simulink library "CRYP_IM_MASTER"  (Simulink 8.6)
settings: Solver=ode45  StartTime=0.0  StopTime=10.0  RelTol=1e-3
libraries: VIS_LIB x14, cdsEpicsOut x10, cdsTP x6, cdsFiltCtrl x4, cdsMuxMatrix x4, CRYP_TM_MASTER x2, cdsFilt x2, KAGRA_UTIL x1, cdsFunctionCall x1
settings Model: Creator=controls  LastModifiedBy=controls

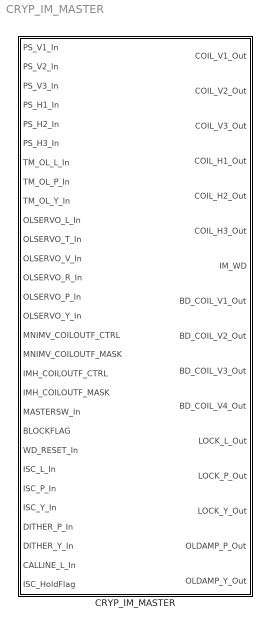
== system CRYP_IM_MASTER ==
  CRYP_IM_MASTER : Subsystem  Description=SIXOSEMSTAGE_FACE_MASTER

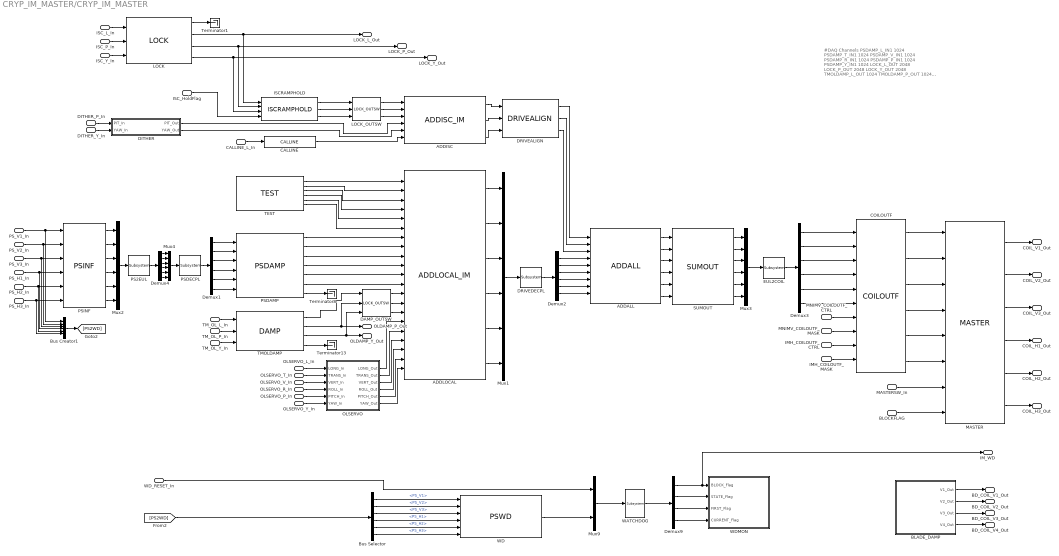
== system CRYP_IM_MASTER/CRYP_IM_MASTER ==
  note: #DAQ Channels
      | PSDAMP_L_IN1 1024
      | PSDAMP_T_IN1 1024
      | PSDAMP_V_IN1 1024
      | PSDAMP_R_IN1 1024
      | PSDAMP_P_IN1 1024
      | PSDAMP_Y_IN1 1024
      | LOCK_L_OUT 2048
      | LOCK_P_OUT 2048
      | LOCK_Y_OUT 2048
      | TMOLDAMP_L_OUT 1024
      | TMOLDAMP_P_OUT 1024
      | TMOLDAMP_Y_OUT 1024
      | PSDAMP_L_OUT 1024
      | PSDAMP_T_OUT 1024
      | PSDAMP_V_OUT 1024
      | PSDAMP_R_OUT 1024
      | PSDAMP_P_OUT 1024
      | PSDAMP_Y_OUT 1024
      | MASTER_OUT_H1 1024
      | MASTER_OUT_H2 1024
      | MASTER_OUT_H3 1024
      | MASTER_OUT_V1 1024
      | MASTER_OUT_V2 1024
      | MASTER_OUT_V3 1024
  PS_V1_In : Inport
  PS_V2_In : Inport  Port=2
  PS_V3_In : Inport  Port=3
  PS_H1_In : Inport  Port=4
  PS_H2_In : Inport  Port=5
  PS_H3_In : Inport  Port=6
  TM_OL_L_In : Inport  Port=7
  TM_OL_P_In : Inport  Port=8
  TM_OL_Y_In : Inport  Port=9
  OLSERVO_L_In : Inport  Port=10
  OLSERVO_T_In : Inport  Port=11
  OLSERVO_V_In : Inport  Port=12
  OLSERVO_R_In : Inport  Port=13
  OLSERVO_P_In : Inport  Port=14
  OLSERVO_Y_In : Inport  Port=15
  MNIMV_COILOUTF_CTRL : Inport  Port=16
  MNIMV_COILOUTF_MASK : Inport  Port=17
  IMH_COILOUTF_CTRL : Inport  Port=18
  IMH_COILOUTF_MASK : Inport  Port=19
  MASTERSW_In : Inport  Port=20
  BLOCKFLAG : Inport  Port=21
  WD_RESET_In : Inport  Port=22
  ISC_L_In : Inport  Port=23
  ISC_P_In : Inport  Port=24
  ISC_Y_In : Inport  Port=25
  DITHER_P_In : Inport  Port=26
  DITHER_Y_In : Inport  Port=27
  CALLINE_L_In : Inport  Port=28
  ISC_HoldFlag : Inport  Port=29
  ADDALL : VIS_LIB/CrypParts/ADDALL
  ADDISC : VIS_LIB/CrypParts/ADDISC_IM
  ADDLOCAL : VIS_LIB/CrypParts/ADDLOCAL_IM
  BLADE_DAMP : Subsystem
  Bus Creator1 : BusCreator  Inputs='PS_V1','PS_V2','PS_V3','PS_H1','PS_H2','PS_H3'
  Bus Selector : BusSelector  OutputSignals=PS_V1,PS_V2,PS_V3,PS_H1,PS_H2,PS_H3
  CALLINE : VIS_LIB/CALLINE
  COILOUTF : VIS_LIB/CRYp Blocks/COILOUTF
  DAMP_OUTSW : CRYP_TM_MASTER/CRYP_TM_MASTER/LOCK_OUTSW
  DITHER : Subsystem
  DRIVEALIGN : VIS_LIB/CrypParts/DRIVEALIGN
  DRIVEDECPL : cdsMuxMatrix/Subsystem  Tag=cdsMuxMatrix  Description=Any size matrix. Inputs and outputs must be connected using Mux and Demux parts.
      settings: AttributesFormatString=%<Tag>
  Demux{1..4} (4 alike) : Demux  Outputs=6
  Demux9 : Demux
  EUL2COIL : cdsMuxMatrix/Subsystem  Tag=cdsMuxMatrix  Description=Any size matrix. Inputs and outputs must be connected using Mux and Demux parts.
      settings: AttributesFormatString=%<Tag>
  ISCRAMPHOLD : KAGRA_UTIL/ISCRAMPHOLD
  LOCK : VIS_LIB/CrypParts/LOCK
  LOCK_OUTSW : CRYP_TM_MASTER/CRYP_TM_MASTER/LOCK_OUTSW
  MASTER : VIS_LIB/CRYp Blocks/MASTER
  Mux{1..4} (4 alike) : Mux  Inputs=6
  Mux9 : Mux  Inputs=2
  OLSERVO : Subsystem
  PS2EUL : cdsMuxMatrix/Subsystem  Tag=cdsMuxMatrix  Description=Any size matrix. Inputs and outputs must be connected using Mux and Demux parts.
      settings: AttributesFormatString=%<Tag>
  PSDAMP : VIS_LIB/CrypParts/PSDAMP
  PSDECPL : cdsMuxMatrix/Subsystem  Tag=cdsMuxMatrix  Description=Any size matrix. Inputs and outputs must be connected using Mux and Demux parts.
      settings: AttributesFormatString=%<Tag>
  PSINF : VIS_LIB/CrypParts/PSINF
  SUMOUT : VIS_LIB/CrypParts/SUMOUT
  TEST : VIS_LIB/CrypParts/TEST
  TMOLDAMP : VIS_LIB/CrypParts/DAMP
  Terminator1 : Terminator
  Terminator13 : Terminator
  Terminator8 : Terminator
  WATCHDOG : cdsFunctionCall/Subsystem  Tag=cdsFunctionCall  Description=inline OSEMWATCHDOG /opt/rtcds/userapps/release/vis/common/src/WATCHDOG.c
      settings: AttributesFormatString=%<Tag>\n%<Description>
  WD : VIS_LIB/CRYp Blocks/PSWD
  WDMON : Subsystem
  COIL_V1_Out : Outport
  COIL_V2_Out : Outport  Port=2
  COIL_V3_Out : Outport  Port=3
  COIL_H1_Out : Outport  Port=4
  COIL_H2_Out : Outport  Port=5
  COIL_H3_Out : Outport  Port=6
  IM_WD : Outport  Port=7
  BD_COIL_V1_Out : Outport  Port=8
  BD_COIL_V2_Out : Outport  Port=9
  BD_COIL_V3_Out : Outport  Port=10
  BD_COIL_V4_Out : Outport  Port=11
  LOCK_L_Out : Outport  Port=12
  LOCK_P_Out : Outport  Port=13
  LOCK_Y_Out : Outport  Port=14
  OLDAMP_P_Out : Outport  Port=15
  OLDAMP_Y_Out : Outport  Port=16
  wires:
  ISC_HoldFlag/1 -> ISCRAMPHOLD/4
  ISCRAMPHOLD/3 -> LOCK_OUTSW/3
  ISCRAMPHOLD/2 -> LOCK_OUTSW/2
  ISCRAMPHOLD/1 -> LOCK_OUTSW/1
  WATCHDOG/1 -> Demux9/1
  Mux9/1 -> WATCHDOG/1
  COILOUTF/3 -> MASTER/3
  COILOUTF/2 -> MASTER/2
  COILOUTF/1 -> MASTER/1
  Demux9/4 -> WDMON/4(CURRENT_Flag)
  Demux9/3 -> WDMON/3(FIRST_Flag)
  Demux9/2 -> WDMON/2(STATE_Flag)
  EUL2COIL/1 -> Demux3/1
  Mux3/1 -> EUL2COIL/1
  MASTER/6 -> COIL_H3_Out/1
  MASTER/5 -> COIL_H2_Out/1
  MASTER/4 -> COIL_H1_Out/1
  MASTER/3 -> COIL_V3_Out/1
  MASTER/2 -> COIL_V2_Out/1
  MASTER/1 -> COIL_V1_Out/1
  [PS2WD] -> Bus Selector/1
  Bus Creator1/1 -> [PS2WD]
  Mux2/1 -> PS2EUL/1
  PSINF/1 -> Mux2/1
  PSINF/2 -> Mux2/2
  PSINF/3 -> Mux2/3
  PSINF/4 -> Mux2/4
  PSINF/5 -> Mux2/5
  PSINF/6 -> Mux2/6
  Demux9/1 -> IM_WD/1, WDMON/1(BLOCK_Flag)
  MASTERSW_In/1 -> MASTER/7
  MNIMV_COILOUTF_CTRL/1 -> COILOUTF/7
  WD/1 -> Mux9/2
  WD_RESET_In/1 -> Mux9/1
  IMH_COILOUTF_CTRL/1 -> COILOUTF/9
  IMH_COILOUTF_MASK/1 -> COILOUTF/10
  PS_V3_In/1 -> Bus Creator1/3, PSINF/3
  PS_H1_In/1 -> PSINF/4, Bus Creator1/4
  PS_H2_In/1 -> Bus Creator1/5, PSINF/5
  PS_H3_In/1 -> Bus Creator1/6, PSINF/6
  PS_V1_In/1 -> Bus Creator1/1, PSINF/1
  PS_V2_In/1 -> Bus Creator1/2, PSINF/2
  MNIMV_COILOUTF_MASK/1 -> COILOUTF/8
  COILOUTF/4 -> MASTER/4
  COILOUTF/5 -> MASTER/5
  COILOUTF/6 -> MASTER/6
  ISC_L_In/1 -> LOCK/1
  ISC_P_In/1 -> LOCK/2
  ISC_Y_In/1 -> LOCK/3
  Bus Selector/6 -> WD/6  "<PS_H3>"
  Bus Selector/1 -> WD/1  "<PS_V1>"
  Bus Selector/2 -> WD/2  "<PS_V2>"
  Bus Selector/3 -> WD/3  "<PS_V3>"
  Bus Selector/4 -> WD/4  "<PS_H1>"
  Bus Selector/5 -> WD/5  "<PS_H2>"
  BLADE_DAMP/1(V1_Out) -> BD_COIL_V1_Out/1
  BLADE_DAMP/2(V2_Out) -> BD_COIL_V2_Out/1
  BLADE_DAMP/3(V3_Out) -> BD_COIL_V3_Out/1
  BLADE_DAMP/4(V4_Out) -> BD_COIL_V4_Out/1
  BLOCKFLAG/1 -> MASTER/8
  Demux3/6 -> COILOUTF/6
  Demux3/5 -> COILOUTF/5
  Demux3/4 -> COILOUTF/4
  Demux3/3 -> COILOUTF/3
  Demux3/2 -> COILOUTF/2
  Demux3/1 -> COILOUTF/1
  Demux1/1 -> PSDAMP/1
  Demux1/2 -> PSDAMP/2
  Demux1/3 -> PSDAMP/3
  Demux1/4 -> PSDAMP/4
  Demux1/5 -> PSDAMP/5
  Demux1/6 -> PSDAMP/6
  PSDAMP/7 -> Terminator8/1
  DITHER/1(PIT_Out) -> ADDISC/4
  DITHER/2(YAW_Out) -> ADDISC/5
  ADDISC/2 -> DRIVEALIGN/2
  ADDISC/1 -> DRIVEALIGN/1
  ADDISC/3 -> DRIVEALIGN/3
  TEST/6 -> ADDLOCAL/6
  TEST/5 -> ADDLOCAL/5
  TEST/4 -> ADDLOCAL/4
  TEST/3 -> ADDLOCAL/3
  TEST/2 -> ADDLOCAL/2
  TEST/1 -> ADDLOCAL/1
  PSDAMP/4 -> ADDLOCAL/10
  PSDAMP/5 -> ADDLOCAL/11
  PSDAMP/6 -> ADDLOCAL/12
  PSDAMP/1 -> ADDLOCAL/7
  PSDAMP/2 -> ADDLOCAL/8
  PSDAMP/3 -> ADDLOCAL/9
  TM_OL_L_In/1 -> TMOLDAMP/1
  TM_OL_P_In/1 -> TMOLDAMP/2
  TM_OL_Y_In/1 -> TMOLDAMP/3
  TMOLDAMP/2 -> OLDAMP_P_Out/1, DAMP_OUTSW/2
  TMOLDAMP/3 -> DAMP_OUTSW/3, OLDAMP_Y_Out/1
  TMOLDAMP/4 -> Terminator13/1
  DRIVEDECPL/1 -> Demux2/1
  Mux1/1 -> DRIVEDECPL/1
  Demux2/5 -> ADDALL/8
  Demux2/2 -> ADDALL/5
  Demux2/3 -> ADDALL/6
  Demux2/6 -> ADDALL/9
  Demux2/1 -> ADDALL/4
  Demux2/4 -> ADDALL/7
  ADDLOCAL/5 -> Mux1/5
  ADDLOCAL/4 -> Mux1/4
  ADDLOCAL/6 -> Mux1/6
  ADDLOCAL/3 -> Mux1/3
  ADDLOCAL/2 -> Mux1/2
  ADDLOCAL/1 -> Mux1/1
  DRIVEALIGN/3 -> ADDALL/3
  DRIVEALIGN/2 -> ADDALL/2
  DRIVEALIGN/1 -> ADDALL/1
  LOCK/1 -> Terminator1/1
  LOCK/4 -> LOCK_Y_Out/1, ISCRAMPHOLD/3
  LOCK/3 -> LOCK_P_Out/1, ISCRAMPHOLD/2
  LOCK/2 -> LOCK_L_Out/1, ISCRAMPHOLD/1
  DITHER_Y_In/1 -> DITHER/2(YAW_In)
  DITHER_P_In/1 -> DITHER/1(PIT_In)
  ADDALL/1 -> SUMOUT/1
  ADDALL/2 -> SUMOUT/2
  ADDALL/3 -> SUMOUT/3
  ADDALL/4 -> SUMOUT/4
  ADDALL/5 -> SUMOUT/5
  ADDALL/6 -> SUMOUT/6
  SUMOUT/1 -> Mux3/1
  SUMOUT/2 -> Mux3/2
  SUMOUT/3 -> Mux3/3
  SUMOUT/4 -> Mux3/4
  SUMOUT/5 -> Mux3/5
  SUMOUT/6 -> Mux3/6
  PSDECPL/1 -> Demux1/1
  PS2EUL/1 -> Demux4/1
  Demux4/1 -> Mux4/1
  Demux4/2 -> Mux4/2
  Demux4/3 -> Mux4/3
  Demux4/4 -> Mux4/4
  Demux4/5 -> Mux4/5
  Demux4/6 -> Mux4/6
  Mux4/1 -> PSDECPL/1
  OLSERVO_L_In/1 -> OLSERVO/1(LONG_In)
  OLSERVO_T_In/1 -> OLSERVO/2(TRANS_In)
  OLSERVO_V_In/1 -> OLSERVO/3(VERT_In)
  OLSERVO_R_In/1 -> OLSERVO/4(ROLL_In)
  OLSERVO_P_In/1 -> OLSERVO/5(PITCH_In)
  OLSERVO_Y_In/1 -> OLSERVO/6(YAW_In)
  OLSERVO/1(LONG_Out) -> ADDLOCAL/16
  OLSERVO/2(TRANS_Out) -> ADDLOCAL/17
  OLSERVO/3(VERT_Out) -> ADDLOCAL/18
  OLSERVO/4(ROLL_Out) -> ADDLOCAL/19
  OLSERVO/5(PITCH_Out) -> ADDLOCAL/20
  OLSERVO/6(YAW_Out) -> ADDLOCAL/21
  LOCK_OUTSW/1 -> ADDISC/1
  LOCK_OUTSW/2 -> ADDISC/2
  LOCK_OUTSW/3 -> ADDISC/3
  DAMP_OUTSW/1 -> ADDLOCAL/13
  DAMP_OUTSW/2 -> ADDLOCAL/14
  DAMP_OUTSW/3 -> ADDLOCAL/15
  TMOLDAMP/1 -> DAMP_OUTSW/1
  CALLINE/1 -> ADDISC/6
  CALLINE_L_In/1 -> CALLINE/1

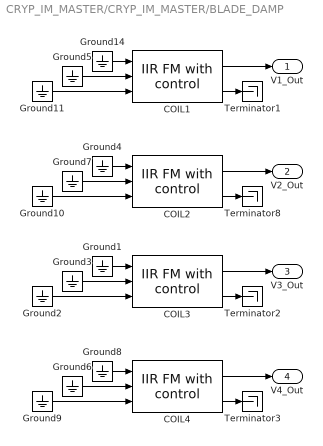
== system CRYP_IM_MASTER/CRYP_IM_MASTER/BLADE_DAMP ==
  COIL1 : cdsFiltCtrl/IIR FM with control  Tag=cdsFiltCtrl  Description=|
      | cdsFiltCntrl is the standard IIR filter module (exactly the same as cdsFilt) but with added control data output 'Ctrl'. Filter module digital signal output appears on the first output, which is called 'Val'. 'Ctrl' output has a bit pattern encoding the state of filter's on/off switches (FM1 through FM10). The bit values are:
      |                                                                                                                                                                                                                                                                                                                                       
      | module 	hex	dec                                                                                                                                                                                                                                                                                                                       
      | -----------------------                                                                                                                                                                                                                                                                                                               
      | FM1	0x20                    32                                                                                                                                                                                                                                                                                                        
      | FM2	0x80                     128                                                                                                                                                                                                                                                                                                      
      | FM3	0x200                   512                                                                                                                                                                                                                                                                                                       
      | FM4	0x800                   2048                                                                                                                                                                                                                                                                                                      
      | FM5	0x2000                 8192                                                                                                                                                                                                                                                                                                       
      | FM6	0x8000                 32768                                                                                                                                                                                                                                                                                                      
      | FM7	0x20000                131072                                                                                                                                                                                                                                                                                                     
      | FM8	0x80000                 524288                                                                                                                                                                                                                                                                                                    
      | FM9	0x200000               2097152                                                                                                                                                                                                                                                                                                    
      | FM10	0x800000               8388608                                                                                                                                                                                                                                                                                                   
      |                                                                                                                                                                                                                                                                                                                                       
      | This bit data can be used to drive some other switches or it can be output using a binary I/O module.
      settings: AttributesFormatString=%<Tag>
  COIL2 : cdsFiltCtrl/IIR FM with control  Tag=cdsFiltCtrl  Description=|
      | cdsFiltCntrl is the standard IIR filter module (exactly the same as cdsFilt) but with added control data output 'Ctrl'. Filter module digital signal output appears on the first output, which is called 'Val'. 'Ctrl' output has a bit pattern encoding the state of filter's on/off switches (FM1 through FM10). The bit values are:
      |                                                                                                                                                                                                                                                                                                                                       
      | module 	hex	dec                                                                                                                                                                                                                                                                                                                       
      | -----------------------                                                                                                                                                                                                                                                                                                               
      | FM1	0x20                    32                                                                                                                                                                                                                                                                                                        
      | FM2	0x80                     128                                                                                                                                                                                                                                                                                                      
      | FM3	0x200                   512                                                                                                                                                                                                                                                                                                       
      | FM4	0x800                   2048                                                                                                                                                                                                                                                                                                      
      | FM5	0x2000                 8192                                                                                                                                                                                                                                                                                                       
      | FM6	0x8000                 32768                                                                                                                                                                                                                                                                                                      
      | FM7	0x20000                131072                                                                                                                                                                                                                                                                                                     
      | FM8	0x80000                 524288                                                                                                                                                                                                                                                                                                    
      | FM9	0x200000               2097152                                                                                                                                                                                                                                                                                                    
      | FM10	0x800000               8388608                                                                                                                                                                                                                                                                                                   
      |                                                                                                                                                                                                                                                                                                                                       
      | This bit data can be used to drive some other switches or it can be output using a binary I/O module.
      settings: AttributesFormatString=%<Tag>
  COIL3 : cdsFiltCtrl/IIR FM with control  Tag=cdsFiltCtrl  Description=|
      | cdsFiltCntrl is the standard IIR filter module (exactly the same as cdsFilt) but with added control data output 'Ctrl'. Filter module digital signal output appears on the first output, which is called 'Val'. 'Ctrl' output has a bit pattern encoding the state of filter's on/off switches (FM1 through FM10). The bit values are:
      |                                                                                                                                                                                                                                                                                                                                       
      | module 	hex	dec                                                                                                                                                                                                                                                                                                                       
      | -----------------------                                                                                                                                                                                                                                                                                                               
      | FM1	0x20                    32                                                                                                                                                                                                                                                                                                        
      | FM2	0x80                     128                                                                                                                                                                                                                                                                                                      
      | FM3	0x200                   512                                                                                                                                                                                                                                                                                                       
      | FM4	0x800                   2048                                                                                                                                                                                                                                                                                                      
      | FM5	0x2000                 8192                                                                                                                                                                                                                                                                                                       
      | FM6	0x8000                 32768                                                                                                                                                                                                                                                                                                      
      | FM7	0x20000                131072                                                                                                                                                                                                                                                                                                     
      | FM8	0x80000                 524288                                                                                                                                                                                                                                                                                                    
      | FM9	0x200000               2097152                                                                                                                                                                                                                                                                                                    
      | FM10	0x800000               8388608                                                                                                                                                                                                                                                                                                   
      |                                                                                                                                                                                                                                                                                                                                       
      | This bit data can be used to drive some other switches or it can be output using a binary I/O module.
      settings: AttributesFormatString=%<Tag>
  COIL4 : cdsFiltCtrl/IIR FM with control  Tag=cdsFiltCtrl  Description=|
      | cdsFiltCntrl is the standard IIR filter module (exactly the same as cdsFilt) but with added control data output 'Ctrl'. Filter module digital signal output appears on the first output, which is called 'Val'. 'Ctrl' output has a bit pattern encoding the state of filter's on/off switches (FM1 through FM10). The bit values are:
      |                                                                                                                                                                                                                                                                                                                                       
      | module 	hex	dec                                                                                                                                                                                                                                                                                                                       
      | -----------------------                                                                                                                                                                                                                                                                                                               
      | FM1	0x20                    32                                                                                                                                                                                                                                                                                                        
      | FM2	0x80                     128                                                                                                                                                                                                                                                                                                      
      | FM3	0x200                   512                                                                                                                                                                                                                                                                                                       
      | FM4	0x800                   2048                                                                                                                                                                                                                                                                                                      
      | FM5	0x2000                 8192                                                                                                                                                                                                                                                                                                       
      | FM6	0x8000                 32768                                                                                                                                                                                                                                                                                                      
      | FM7	0x20000                131072                                                                                                                                                                                                                                                                                                     
      | FM8	0x80000                 524288                                                                                                                                                                                                                                                                                                    
      | FM9	0x200000               2097152                                                                                                                                                                                                                                                                                                    
      | FM10	0x800000               8388608                                                                                                                                                                                                                                                                                                   
      |                                                                                                                                                                                                                                                                                                                                       
      | This bit data can be used to drive some other switches or it can be output using a binary I/O module.
      settings: AttributesFormatString=%<Tag>
  Ground{1..11,14} (12 alike) : Ground
  Terminator{1..3,8} (4 alike) : Terminator
  V1_Out : Outport
  V2_Out : Outport  Port=2
  V3_Out : Outport  Port=3
  V4_Out : Outport  Port=4
  wires:
  COIL1/1 -> V1_Out/1
  COIL2/1 -> V2_Out/1
  COIL3/1 -> V3_Out/1
  COIL4/1 -> V4_Out/1
  Ground14/1 -> COIL1/1
  Ground5/1 -> COIL1/2
  Ground11/1 -> COIL1/3
  Ground4/1 -> COIL2/1
  Ground7/1 -> COIL2/2
  Ground10/1 -> COIL2/3
  Ground1/1 -> COIL3/1
  Ground3/1 -> COIL3/2
  Ground2/1 -> COIL3/3
  Ground8/1 -> COIL4/1
  Ground6/1 -> COIL4/2
  Ground9/1 -> COIL4/3
  COIL1/2 -> Terminator1/1
  COIL2/2 -> Terminator8/1
  COIL3/2 -> Terminator2/1
  COIL4/2 -> Terminator3/1

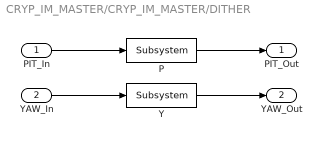
== system CRYP_IM_MASTER/CRYP_IM_MASTER/DITHER ==
  PIT_In : Inport
  YAW_In : Inport  Port=2
  P : cdsFilt/Subsystem  Tag=cdsFilt  Description=|
      | Purpose:                                                                                                                                                                                                                                  
      | Standard CDS IIR filter module.                                                                                                                                                                                                           
      |                                                                                                                                                                                                                                           
      | Operation:                                                                                                                                                                                                                                
      | Consists of 10 second order section IIR filters, plus a ramped gain stage. In FE code, also provides pre-defined test points and excitation channel inputs. The filter coefficients are defined in the LIGO system using the 'foton' tool.
      |                                                                                                                                                                                                                                           
      | Usage:                                                                                                                                                                                                                                    
      | Name the part with the desired filter module name.
      settings: AttributesFormatString=%<Tag>
  Y : cdsFilt/Subsystem  Tag=cdsFilt  Description=|
      | Purpose:                                                                                                                                                                                                                                  
      | Standard CDS IIR filter module.                                                                                                                                                                                                           
      |                                                                                                                                                                                                                                           
      | Operation:                                                                                                                                                                                                                                
      | Consists of 10 second order section IIR filters, plus a ramped gain stage. In FE code, also provides pre-defined test points and excitation channel inputs. The filter coefficients are defined in the LIGO system using the 'foton' tool.
      |                                                                                                                                                                                                                                           
      | Usage:                                                                                                                                                                                                                                    
      | Name the part with the desired filter module name.
      settings: AttributesFormatString=%<Tag>
  PIT_Out : Outport
  YAW_Out : Outport  Port=2
  wires:
  PIT_In/1 -> P/1
  Y/1 -> YAW_Out/1
  YAW_In/1 -> Y/1
  P/1 -> PIT_Out/1

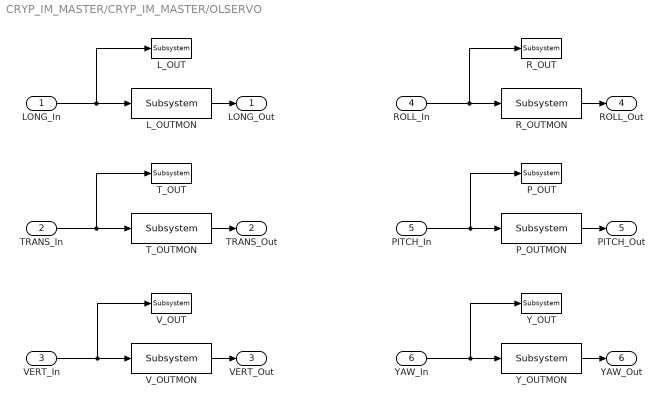
== system CRYP_IM_MASTER/CRYP_IM_MASTER/OLSERVO ==
  LONG_In : Inport
  TRANS_In : Inport  Port=2
  VERT_In : Inport  Port=3
  ROLL_In : Inport  Port=4
  PITCH_In : Inport  Port=5
  YAW_In : Inport  Port=6
  L_OUT : cdsTP/Subsystem  Tag=Test Point
      settings: AttributesFormatString=%<Tag>
  L_OUTMON : cdsEpicsOut/Subsystem  Tag=cdsEpicsOutput  Description=|
      | Purpose:                                          
      | Output a FE signal to an EPICS channel.           
      |                                                   
      | Operation:                                        
      | Takes input value and passes it to EPICS record.  
      |                                                   
      | Usage:                                            
      | Name the part with the desired EPICS rrecord name.
      settings: AttributesFormatString=%<Tag>
  P_OUT : cdsTP/Subsystem  Tag=Test Point
      settings: AttributesFormatString=%<Tag>
  P_OUTMON : cdsEpicsOut/Subsystem  Tag=cdsEpicsOutput  Description=|
      | Purpose:                                          
      | Output a FE signal to an EPICS channel.           
      |                                                   
      | Operation:                                        
      | Takes input value and passes it to EPICS record.  
      |                                                   
      | Usage:                                            
      | Name the part with the desired EPICS rrecord name.
      settings: AttributesFormatString=%<Tag>
  R_OUT : cdsTP/Subsystem  Tag=Test Point
      settings: AttributesFormatString=%<Tag>
  R_OUTMON : cdsEpicsOut/Subsystem  Tag=cdsEpicsOutput  Description=|
      | Purpose:                                          
      | Output a FE signal to an EPICS channel.           
      |                                                   
      | Operation:                                        
      | Takes input value and passes it to EPICS record.  
      |                                                   
      | Usage:                                            
      | Name the part with the desired EPICS rrecord name.
      settings: AttributesFormatString=%<Tag>
  T_OUT : cdsTP/Subsystem  Tag=Test Point
      settings: AttributesFormatString=%<Tag>
  T_OUTMON : cdsEpicsOut/Subsystem  Tag=cdsEpicsOutput  Description=|
      | Purpose:                                          
      | Output a FE signal to an EPICS channel.           
      |                                                   
      | Operation:                                        
      | Takes input value and passes it to EPICS record.  
      |                                                   
      | Usage:                                            
      | Name the part with the desired EPICS rrecord name.
      settings: AttributesFormatString=%<Tag>
  V_OUT : cdsTP/Subsystem  Tag=Test Point
      settings: AttributesFormatString=%<Tag>
  V_OUTMON : cdsEpicsOut/Subsystem  Tag=cdsEpicsOutput  Description=|
      | Purpose:                                          
      | Output a FE signal to an EPICS channel.           
      |                                                   
      | Operation:                                        
      | Takes input value and passes it to EPICS record.  
      |                                                   
      | Usage:                                            
      | Name the part with the desired EPICS rrecord name.
      settings: AttributesFormatString=%<Tag>
  Y_OUT : cdsTP/Subsystem  Tag=Test Point
      settings: AttributesFormatString=%<Tag>
  Y_OUTMON : cdsEpicsOut/Subsystem  Tag=cdsEpicsOutput  Description=|
      | Purpose:                                          
      | Output a FE signal to an EPICS channel.           
      |                                                   
      | Operation:                                        
      | Takes input value and passes it to EPICS record.  
      |                                                   
      | Usage:                                            
      | Name the part with the desired EPICS rrecord name.
      settings: AttributesFormatString=%<Tag>
  LONG_Out : Outport
  TRANS_Out : Outport  Port=2
  VERT_Out : Outport  Port=3
  ROLL_Out : Outport  Port=4
  PITCH_Out : Outport  Port=5
  YAW_Out : Outport  Port=6
  wires:
  L_OUTMON/1 -> LONG_Out/1
  LONG_In/1 -> L_OUT/1, L_OUTMON/1
  T_OUTMON/1 -> TRANS_Out/1
  TRANS_In/1 -> T_OUT/1, T_OUTMON/1
  V_OUTMON/1 -> VERT_Out/1
  R_OUTMON/1 -> ROLL_Out/1
  ROLL_In/1 -> R_OUT/1, R_OUTMON/1
  VERT_In/1 -> V_OUT/1, V_OUTMON/1
  P_OUTMON/1 -> PITCH_Out/1
  PITCH_In/1 -> P_OUT/1, P_OUTMON/1
  Y_OUTMON/1 -> YAW_Out/1
  YAW_In/1 -> Y_OUT/1, Y_OUTMON/1

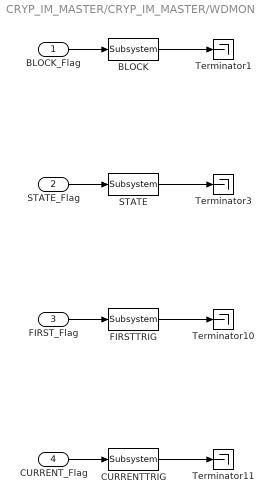
== system CRYP_IM_MASTER/CRYP_IM_MASTER/WDMON ==
  BLOCK_Flag : Inport
  STATE_Flag : Inport  Port=2
  FIRST_Flag : Inport  Port=3
  CURRENT_Flag : Inport  Port=4
  BLOCK : cdsEpicsOut/Subsystem  Tag=cdsEpicsOutput  Description="field(PREC,\"3\")"
      settings: AttributesFormatString=%<Tag>
  CURRENTTRIG : cdsEpicsOut/Subsystem  Tag=cdsEpicsOutput  Description="field(PREC,\"3\")"
      settings: AttributesFormatString=%<Tag>
  FIRSTTRIG : cdsEpicsOut/Subsystem  Tag=cdsEpicsOutput  Description="field(PREC,\"3\")"
      settings: AttributesFormatString=%<Tag>
  STATE : cdsEpicsOut/Subsystem  Tag=cdsEpicsOutput  Description="field(PREC,\"3\")"
      settings: AttributesFormatString=%<Tag>
  Terminator{1,3,10..11} (4 alike) : Terminator
  wires:
  STATE/1 -> Terminator3/1
  BLOCK/1 -> Terminator1/1
  BLOCK_Flag/1 -> BLOCK/1
  FIRSTTRIG/1 -> Terminator10/1
  CURRENTTRIG/1 -> Terminator11/1
  CURRENT_Flag/1 -> CURRENTTRIG/1
  FIRST_Flag/1 -> FIRSTTRIG/1
  STATE_Flag/1 -> STATE/1
